simulink model "AariaHIABTorqueR2017a"  (R2017a)
settings: Solver=VariableStepAuto  StartTime=0.0  StopTime=inf  FixedStep=0.1  RelTol=1e-3  EnableMultiTasking=on
model workspace (MATLAB code in the model file):
  | my_a =1;
undefined symbols (not defined in the file or in its folder): AARIAENV, AARIAMAN, AARIASEN, Camera, sensor, Source_TS, X, Y, Z
libraries: sm_lib x350, nesl_utility x205, dspmathops x80, simulink x66, powerlib_meascontrol x3, vrlib x2, aerolibanimutils x1, aerolibutil x1
(part 4 of 9)

== system AariaHIABTorqueR2017a/Subsystem/grab_check_cam above angled down ==
  note: compares spherical coordinates from tool to camera and camera to object (doesn't work always)
  note: compares spherical coordinates from camera to and camera to object
  CamObjSph : Inport
  ObjPose : Inport  Port=2
  TipCamSph : Inport  Port=3
  Logical Operator : Logic  AllPortsSameDT=off  OutDataTypeStr=boolean
  Subsystem : Subsystem
  Sum : Sum
  orientation match : Subsystem  Commented=on
  orientation match1 : Subsystem
  pose match : Subsystem
  grab ok : Outport
  pose ok : Outport  Port=2
  orientation ok : Outport  Port=3
  Bonus : Outport  Port=4  OutDataTypeStr=double
  wires:
  TipCamSph/1 -> orientation match1/1(TipCam)
  Subsystem/1(TipObjPose) -> pose match/1(Obj_pose)
  ObjPose/1 -> Subsystem/1(CamObj)
  CamObjSph/1 -> orientation match1/2(CamObj)
  pose match/1(grab_pose_ok) -> pose ok/1, Logical Operator/1
  Logical Operator/1 -> grab ok/1
  orientation match1/2(Orient_penalty) -> Sum/2
  pose match/2(PoseBonus) -> Sum/1
  Sum/1 -> Bonus/1
  orientation match1/1(Out1) -> orientation ok/1, Logical Operator/2

== system AariaHIABTorqueR2017a/Subsystem2/Subsystem1 ==
  Trigger : TriggerPort  VariantControl=Variant  PortDimensions=1
  Constant : Constant
  Constant1 : Constant  Value=0
  Memory : Memory  InheritSampleTime=on
  Switch : Switch  Criteria=u2 > Threshold
  Out1 : Outport
  wires:
  Constant/1 -> Switch/3
  Switch/1 -> Out1/1, Memory/1
  Memory/1 -> Switch/2
  Constant1/1 -> Switch/1

== system AariaHIABTorqueR2017a/Tool/IMU Tool ==
  Sensor Module1 : Subsystem  mask{nL=nL, nS=1}
      mask prompts: nL "Link Number"; nS "Sensor ID of that link"
      mask DialogControl DescGroupVar Prompt: Virtual IMU
      mask DialogControl DescTextVar Prompt: Measures Connected Body's acceleration and angular velocity in the given point
      mask DialogControl Control2 Prompt: The following numbers defines the corresponding numbers for this sensor to read from the parameters file
  Body Coord : PMIOPort  Port=1  Side=Left
  Reference Coord : PMIOPort  Port=2  Side=Left
  Out1 : Outport
  Out2 : Outport  Port=2
  Out3 : Outport  Port=3
  Out4 : Outport  Port=4
  wires:
  Sensor Module1/3(Out2) -> Out3/1
  Sensor Module1/2(Out4) -> Out2/1
  Sensor Module1/4(Out3) -> Out4/1
  Sensor Module1/1(Out5) -> Out1/1
  connections:
  Sensor Module1/LConn2 -- Reference Coord/RConn1
  Sensor Module1/LConn1 -- Body Coord/RConn1

== system AariaHIABTorqueR2017a/Tool/IMU Tool1 ==
  Sensor Module1 : Subsystem  mask{nL=nL, nS=1}
      mask prompts: nL "Link Number"; nS "Sensor ID of that link"
      mask DialogControl DescGroupVar Prompt: Virtual IMU
      mask DialogControl DescTextVar Prompt: Measures Connected Body's acceleration and angular velocity in the given point
      mask DialogControl Control2 Prompt: The following numbers defines the corresponding numbers for this sensor to read from the parameters file
  Body Coord : PMIOPort  Port=1  Side=Left
  Reference Coord : PMIOPort  Port=2  Side=Left
  Out1 : Outport
  Out2 : Outport  Port=2
  Out3 : Outport  Port=3
  Out4 : Outport  Port=4
  wires:
  Sensor Module1/1(Out5) -> Out1/1
  Sensor Module1/4(Out3) -> Out4/1
  Sensor Module1/2(Out4) -> Out2/1
  Sensor Module1/3(Out2) -> Out3/1
  connections:
  Sensor Module1/LConn1 -- Body Coord/RConn1
  Sensor Module1/LConn2 -- Reference Coord/RConn1

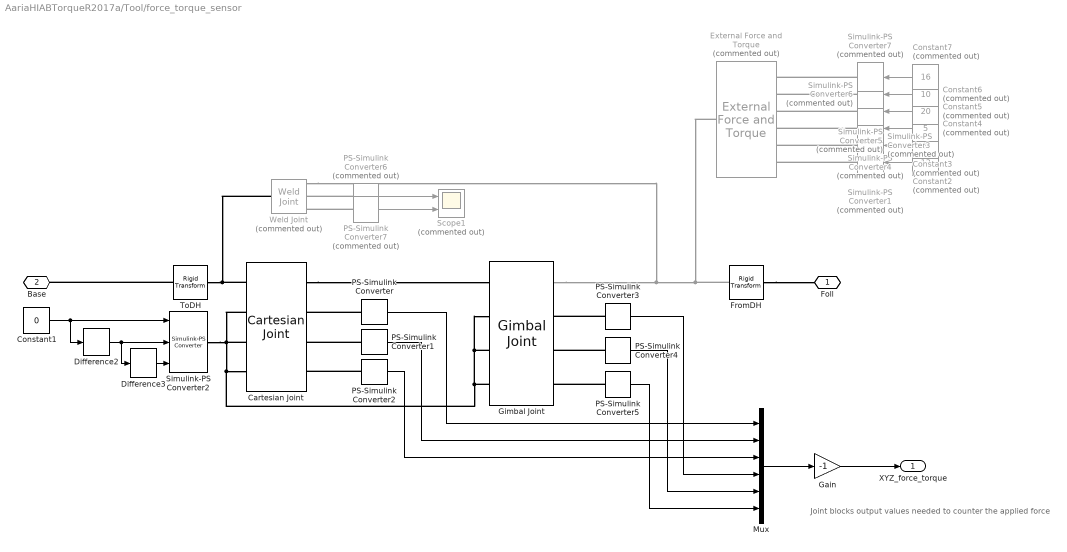
== system AariaHIABTorqueR2017a/Tool/force_torque_sensor ==
  note: Joint blocks output values needed to counter the applied force
  Cartesian Joint : sm_lib/Joints/Cartesian Joint  SenseConstraintForce=off  SenseConstraintForceX=off  SenseConstraintForceY=off  SenseConstraintForceZ=off  SenseConstraintTorque=off  SenseConstraintTorqueX=off  SenseConstraintTorqueY=off  SenseConstraintTorqueZ=off  SenseTotalForce=off  SenseTotalForceX=off  SenseTotalForceY=off  SenseTotalForceZ=off  SenseTotalTorque=off  SenseTotalTorqueX=off  SenseTotalTorqueY=off  SenseTotalTorqueZ=off  CompositeWrenchDir=FollowerOnBase  CompositeWrenchFrame=BaseFrame  PxEquilibriumPosition=0  PxEquilibriumPositionUnits=m  PxSpringStiffness=0  PxSpringStiffnessUnits=N/m  PxDampingCoefficient=0  PxDampingCoefficientUnits=N/(m/s)  PxTorqueActuationMode=ComputedTorque  PxMotionActuationMode=InputMotion  PxSensePosition=off  PxSenseVelocity=off  PxSenseAcceleration=off  PxSenseTorqueForce=on  PxPositionTargetSpecify=off  PxPositionTargetPriority=High  PxPositionTargetValue=0  PxPositionTargetValueUnits=m  PxVelocityTargetSpecify=off  PxVelocityTargetPriority=High  PxVelocityTargetValue=0  PxVelocityTargetValueUnits=m/s  PyEquilibriumPosition=0  PyEquilibriumPositionUnits=m  PySpringStiffness=0  PySpringStiffnessUnits=N/m  PyDampingCoefficient=0  PyDampingCoefficientUnits=N/(m/s)  PyTorqueActuationMode=ComputedTorque  PyMotionActuationMode=InputMotion  PySensePosition=off  PySenseVelocity=off  PySenseAcceleration=off  PySenseTorqueForce=on  PyPositionTargetSpecify=off  PyPositionTargetPriority=High  PyPositionTargetValue=0  PyPositionTargetValueUnits=m  PyVelocityTargetSpecify=off  PyVelocityTargetPriority=High  PyVelocityTargetValue=0  PyVelocityTargetValueUnits=m/s  PzEquilibriumPosition=0  PzEquilibriumPositionUnits=m  PzSpringStiffness=0  PzSpringStiffnessUnits=N/m  PzDampingCoefficient=0  PzDampingCoefficientUnits=N/(m/s)  PzTorqueActuationMode=ComputedTorque  PzMotionActuationMode=InputMotion  PzSensePosition=off  PzSenseVelocity=off  PzSenseAcceleration=off  PzSenseTorqueForce=on  PzPositionTargetSpecify=off  PzPositionTargetPriority=High  PzPositionTargetValue=0  PzPositionTargetValueUnits=m  PzVelocityTargetSpecify=off  PzVelocityTargetPriority=High  PzVelocityTargetValue=0  PzVelocityTargetValueUnits=m/s
  Constant1 : Constant  Value=0
  Constant2 : Constant  Commented=on  Value=13
  Constant3 : Constant  Commented=on
  Constant4 : Constant  Commented=on  Value=5
  Constant5 : Constant  Commented=on  Value=20
  Constant6 : Constant  Commented=on  Value=10
  Constant7 : Constant  Commented=on  Value=16
  Difference2 : simulink/Discrete/Difference  ICPrevInput=0.0  OutMin=[]  OutMax=[]  OutDataType=fixdt(1, 16)  OutScaling=2^-10  DoSatur=off
  Difference3 : simulink/Discrete/Difference  ICPrevInput=0.0  OutMin=[]  OutMax=[]  OutDataType=fixdt(1, 16)  OutScaling=2^-10  DoSatur=off
  External Force and Torque : sm_lib/Forces and Torques/External Force and Torque  Commented=on  ForceResolutionFrame=AttachedFrame  EnableForceX=on  EnableForceY=on  EnableForceZ=on  EnableForce=off  TorqueResolutionFrame=AttachedFrame  EnableTorqueX=on  EnableTorqueY=on  EnableTorqueZ=on  EnableTorque=off
  FromDH : sm_lib/Frames and Transforms/Rigid Transform  TranslationMethod=None  TranslationStandardOffset=0  TranslationLengthUnit=m  TranslationStandardAxis=+Z  TranslationCartesianOffset=[0 0 0]  TranslationROffset=0  TranslationROffsetUnits=m  TranslationZOffset=0  TranslationZOffsetUnits=m  TranslationThetaOffset=0  TranslationThetaOffsetUnits=deg  RotationMethod=RotationMatrix  RotationAngleUnits=deg  RotationStandardAxis=+Z  RotationAngle=0.0  RotationArbitraryAxis=[0 0 1]  FollAlignAxisA=+X  BaseAlignAxisA=+Y  FollAlignAxisB=+Y  BaseAlignAxisB=+Z  RotationSequenceAxes=FollowerAxes  RotationSequence=XYX  RotationSequenceAngles=[0 0 0]  RotationSequenceAnglesUnits=deg  RotationMatrix=AARIAMAN.L(Link_number).toDH'
  Gain : Gain  Gain=-1
  Gimbal Joint : sm_lib/Joints/Gimbal Joint  SenseConstraintForce=off  SenseConstraintForceX=off  SenseConstraintForceY=off  SenseConstraintForceZ=off  SenseConstraintTorque=off  SenseConstraintTorqueX=off  SenseConstraintTorqueY=off  SenseConstraintTorqueZ=off  SenseTotalForce=off  SenseTotalForceX=off  SenseTotalForceY=off  SenseTotalForceZ=off  SenseTotalTorque=off  SenseTotalTorqueX=off  SenseTotalTorqueY=off  SenseTotalTorqueZ=off  CompositeWrenchDir=FollowerOnBase  CompositeWrenchFrame=BaseFrame  RxEquilibriumPosition=0  RxEquilibriumPositionUnits=deg  RxSpringStiffness=0  RxSpringStiffnessUnits=N*m/deg  RxDampingCoefficient=0  RxDampingCoefficientUnits=N*m/(deg/s)  RxTorqueActuationMode=ComputedTorque  RxMotionActuationMode=InputMotion  RxSensePosition=off  RxSenseVelocity=off  RxSenseAcceleration=off  RxSenseTorqueForce=on  RxPositionTargetSpecify=off  RxPositionTargetPriority=High  RxPositionTargetValue=0  RxPositionTargetValueUnits=deg  RxVelocityTargetSpecify=off  RxVelocityTargetPriority=High  RxVelocityTargetValue=0  RxVelocityTargetValueUnits=deg/s  RyEquilibriumPosition=0  RyEquilibriumPositionUnits=deg  RySpringStiffness=0  RySpringStiffnessUnits=N*m/deg  RyDampingCoefficient=0  RyDampingCoefficientUnits=N*m/(deg/s)  RyTorqueActuationMode=ComputedTorque  RyMotionActuationMode=InputMotion  RySensePosition=off  RySenseVelocity=off  RySenseAcceleration=off  RySenseTorqueForce=on  RyPositionTargetSpecify=off  RyPositionTargetPriority=High  RyPositionTargetValue=0  RyPositionTargetValueUnits=deg  RyVelocityTargetSpecify=off  RyVelocityTargetPriority=High  RyVelocityTargetValue=0  RyVelocityTargetValueUnits=deg/s  RzEquilibriumPosition=0  RzEquilibriumPositionUnits=deg  RzSpringStiffness=0  RzSpringStiffnessUnits=N*m/deg  RzDampingCoefficient=0  RzDampingCoefficientUnits=N*m/(deg/s)  RzTorqueActuationMode=ComputedTorque  RzMotionActuationMode=InputMotion  RzSensePosition=off  RzSenseVelocity=off  RzSenseAcceleration=off  RzSenseTorqueForce=on  RzPositionTargetSpecify=off  RzPositionTargetPriority=High  RzPositionTargetValue=0  RzPositionTargetValueUnits=deg  RzVelocityTargetSpecify=off  RzVelocityTargetPriority=High  RzVelocityTargetValue=0  RzVelocityTargetValueUnits=deg/s
      settings: SourceProductName=Simscape Multibody
  Mux : Mux  Inputs=6
  PS-Simulink Converter{,1..5} (6 alike) : nesl_utility/PS-Simulink Converter  PhysicalDomain=network_engine_domain  SubClassName=ps_output  LeftPortType=input  RightPortType=output  PseudoPeriodic=off  Frequencies=[]  Unit=1  AffineConversion=off
  PS-Simulink Converter6 : nesl_utility/PS-Simulink Converter  Commented=on  PhysicalDomain=network_engine_domain  SubClassName=ps_output  LeftPortType=input  RightPortType=output  PseudoPeriodic=off  Frequencies=[]  Unit=1  AffineConversion=off
  PS-Simulink Converter7 : nesl_utility/PS-Simulink Converter  Commented=on  PhysicalDomain=network_engine_domain  SubClassName=ps_output  LeftPortType=input  RightPortType=output  PseudoPeriodic=off  Frequencies=[]  Unit=1  AffineConversion=off
  Scope1 : Scope  Commented=on  NumInputPorts=2
  Simulink-PS Converter{1,3..7} (6 alike) : nesl_utility/Simulink-PS Converter  Commented=on  PhysicalDomain=network_engine_domain  SubClassName=ps_input  LeftPortType=input  RightPortType=output  PseudoPeriodic=off  Frequencies=[]  NoiseDistribution=none  NoiseParameters=[]  Unit=1  AffineConversion=off  FilteringAndDerivatives=provide  SimscapeFilterOrder=1  InputFilterTimeConstant=0.001  UdotUserProvided=0
  Simulink-PS Converter2 : nesl_utility/Simulink-PS Converter  PhysicalDomain=network_engine_domain  SubClassName=ps_input  LeftPortType=input  RightPortType=output  PseudoPeriodic=off  Frequencies=[]  NoiseDistribution=none  NoiseParameters=[]  Unit=1  AffineConversion=off  FilteringAndDerivatives=provide  SimscapeFilterOrder=1  InputFilterTimeConstant=0.001  UdotUserProvided=2
  ToDH : sm_lib/Frames and Transforms/Rigid Transform  TranslationMethod=None  TranslationStandardOffset=0  TranslationLengthUnit=m  TranslationStandardAxis=+Z  TranslationCartesianOffset=[0 0 0]  TranslationROffset=0  TranslationROffsetUnits=m  TranslationZOffset=0  TranslationZOffsetUnits=m  TranslationThetaOffset=0  TranslationThetaOffsetUnits=deg  RotationMethod=RotationMatrix  RotationAngleUnits=deg  RotationStandardAxis=+Z  RotationAngle=0.0  RotationArbitraryAxis=[0 0 1]  FollAlignAxisA=+X  BaseAlignAxisA=+Y  FollAlignAxisB=+Y  BaseAlignAxisB=+Z  RotationSequenceAxes=FollowerAxes  RotationSequence=XYX  RotationSequenceAngles=[0 0 0]  RotationSequenceAnglesUnits=deg  RotationMatrix=AARIAMAN.L(Link_number).toDH
  Weld Joint : sm_lib/Joints/Weld Joint  Commented=on  SenseConstraintForce=on  SenseConstraintForceX=off  SenseConstraintForceY=off  SenseConstraintForceZ=off  SenseConstraintTorque=on  SenseConstraintTorqueX=off  SenseConstraintTorqueY=off  SenseConstraintTorqueZ=off  SenseTotalForce=off  SenseTotalForceX=off  SenseTotalForceY=off  SenseTotalForceZ=off  SenseTotalTorque=off  SenseTotalTorqueX=off  SenseTotalTorqueY=off  SenseTotalTorqueZ=off  CompositeWrenchDir=FollowerOnBase  CompositeWrenchFrame=BaseFrame
  Foll : PMIOPort  Port=1  Side=Right
  Base : PMIOPort  Port=2  Side=Left
  XYZ_force_torque : Outport
  wires:
  Constant1/1 -> Difference2/1, Simulink-PS Converter2/1
  Difference2/1 -> Difference3/1, Simulink-PS Converter2/2
  Difference3/1 -> Simulink-PS Converter2/3
  Constant2/1 -> Simulink-PS Converter1/1
  PS-Simulink Converter/1 -> Mux/1
  PS-Simulink Converter1/1 -> Mux/2
  PS-Simulink Converter2/1 -> Mux/3
  PS-Simulink Converter3/1 -> Mux/4
  PS-Simulink Converter4/1 -> Mux/5
  PS-Simulink Converter5/1 -> Mux/6
  Mux/1 -> Gain/1
  Constant3/1 -> Simulink-PS Converter3/1
  Constant4/1 -> Simulink-PS Converter4/1
  Constant5/1 -> Simulink-PS Converter5/1
  Constant6/1 -> Simulink-PS Converter6/1
  Constant7/1 -> Simulink-PS Converter7/1
  Gain/1 -> XYZ_force_torque/1
  PS-Simulink Converter7/1 -> Scope1/2
  PS-Simulink Converter6/1 -> Scope1/1
  connections:
  Simulink-PS Converter2/RConn1 -- Gimbal Joint/LConn4 -- Gimbal Joint/LConn3 -- Gimbal Joint/LConn2 -- Cartesian Joint/LConn4 -- Cartesian Joint/LConn3 -- Cartesian Joint/LConn2
  PS-Simulink Converter4/LConn1 -- Gimbal Joint/RConn3
  PS-Simulink Converter5/LConn1 -- Gimbal Joint/RConn4
  PS-Simulink Converter3/LConn1 -- Gimbal Joint/RConn2
  ToDH/LConn1 -- Base/RConn1
  PS-Simulink Converter2/LConn1 -- Cartesian Joint/RConn4
  PS-Simulink Converter/LConn1 -- Cartesian Joint/RConn2
  PS-Simulink Converter1/LConn1 -- Cartesian Joint/RConn3
  External Force and Torque/RConn1 -- FromDH/LConn1 -- Weld Joint/RConn1 -- Gimbal Joint/RConn1
  Simulink-PS Converter1/RConn1 -- External Force and Torque/LConn6
  Cartesian Joint/RConn1 -- Gimbal Joint/LConn1
  Cartesian Joint/LConn1 -- ToDH/RConn1 -- Weld Joint/LConn1
  FromDH/RConn1 -- Foll/RConn1
  Simulink-PS Converter3/RConn1 -- External Force and Torque/LConn5
  Simulink-PS Converter4/RConn1 -- External Force and Torque/LConn4
  Simulink-PS Converter5/RConn1 -- External Force and Torque/LConn3
  Simulink-PS Converter6/RConn1 -- External Force and Torque/LConn2
  Simulink-PS Converter7/RConn1 -- External Force and Torque/LConn1
  PS-Simulink Converter6/LConn1 -- Weld Joint/RConn2
  PS-Simulink Converter7/LConn1 -- Weld Joint/RConn3

== system AariaHIABTorqueR2017a/Tool Sensors/Camera sensor ==
  Gain : Gain  Gain=0
  Mux : Mux  Inputs=3
  Mux1 : Mux  Inputs=3
  PS-Simulink Converter{2..8} (7 alike) : nesl_utility/PS-Simulink Converter  PhysicalDomain=network_engine_domain  SubClassName=ps_output  LeftPortType=input  RightPortType=output  PseudoPeriodic=off  Frequencies=[]  Unit=1  AffineConversion=off
  Sum1 : Sum  Inputs=|++
  Sum2 : Sum  Inputs=++|
  Sum3 : Sum  Inputs=++|
  Transform Sensor : sm_lib/Frames and Transforms/Transform Sensor  MeasurementFrame=Base  SenseAngle=off  SenseAxis=off  SenseAngle1=off  SenseAngle2=off  SenseAngle3=off  SenseQ=off  SenseR=on  SenseOmegaX=off  SenseOmegaY=off  SenseOmegaZ=off  SenseOmega1=off  SenseOmega2=off  SenseOmega3=off  SenseQDot=off  SenseRDot=off  SenseAlphaX=off  SenseAlphaY=off  SenseAlphaZ=off  SenseAlpha1=off  SenseAlpha2=off  SenseAlpha3=off  SenseQDDot=off  SenseRDDot=off  SenseX=on  SenseY=on  SenseZ=on  SenseRad=off  SenseAzim=on  SenseDist=on  SenseInc=on  SenseXDot=off  SenseYDot=off  SenseZDot=off  SenseRadDot=off  SenseAzimDot=off  SenseDistDot=off  SenseIncDot=off  SenseXDDot=off  SenseYDDot=off  SenseZDDot=off  SenseRadDDot=off  SenseAzimDDot=off  SenseDistDDot=off  SenseIncDDot=off
  coord_sens : sm_lib/Body Elements/Graphic  GraphicType=Marker  MarkerShape=Frame  MarkerSize=AARIAMAN.vis.coord_sizeS  GraphicVisPropType=SimpleVisualProperties  GraphicDiffuseColor=AARIAMAN.vis.col_s  GraphicSpecularColor=[0.5 0.5 0.5 1.0]  GraphicAmbientColor=[0.15 0.15 0.15 1.0]  GraphicEmissiveColor=[0.0 0.0 0.0 1.0]  GraphicShininess=75  GraphicOpacity=AARIAMAN.vis.opacity_s
      settings: SourceProductName=Simscape Multibody
  omega_noise : Subsystem  Commented=on
  placeholder noise 3 : Subsystem
  placeholder noise1 : Subsystem
  placeholder noise2 : Subsystem
  Body Frame : PMIOPort  Port=1  Side=Left
  Reference Frame : PMIOPort  Port=2  Side=Left
  Out3 : Outport
  Out1 : Outport  Port=2
  Out2 : Outport  Port=3
  wires:
  Sum2/1 -> Out1/1  "cartesian"
  PS-Simulink Converter8/1 -> Sum3/2  "R_actual"
  PS-Simulink Converter7/1 -> Mux1/3
  PS-Simulink Converter5/1 -> Mux1/1
  PS-Simulink Converter6/1 -> Mux1/2
  Mux/1 -> Sum2/2  "cartesian"
  PS-Simulink Converter4/1 -> Mux/3
  PS-Simulink Converter2/1 -> Mux/1
  PS-Simulink Converter3/1 -> Mux/2
  Mux1/1 -> Sum1/1  "spherical"
  Sum3/1 -> Out3/1  "rotation"
  placeholder noise2/1(noise) -> Sum3/1
  placeholder noise 3/1(noise) -> Gain/1
  Sum1/1 -> Out2/1  "spherical"
  placeholder noise1/1(noise) -> Sum2/1
  Gain/1 -> Sum1/2
  connections:
  Transform Sensor/RConn7 -- PS-Simulink Converter6/LConn1
  Transform Sensor/RConn8 -- PS-Simulink Converter7/LConn1
  PS-Simulink Converter8/LConn1 -- Transform Sensor/RConn2
  Transform Sensor/RConn6 -- PS-Simulink Converter5/LConn1
  Transform Sensor/RConn5 -- PS-Simulink Converter4/LConn1
  Transform Sensor/LConn1 -- Reference Frame/RConn1
  Transform Sensor/RConn4 -- PS-Simulink Converter3/LConn1
  Transform Sensor/RConn3 -- PS-Simulink Converter2/LConn1
  coord_sens/RConn1 -- Body Frame/RConn1 -- Transform Sensor/RConn1

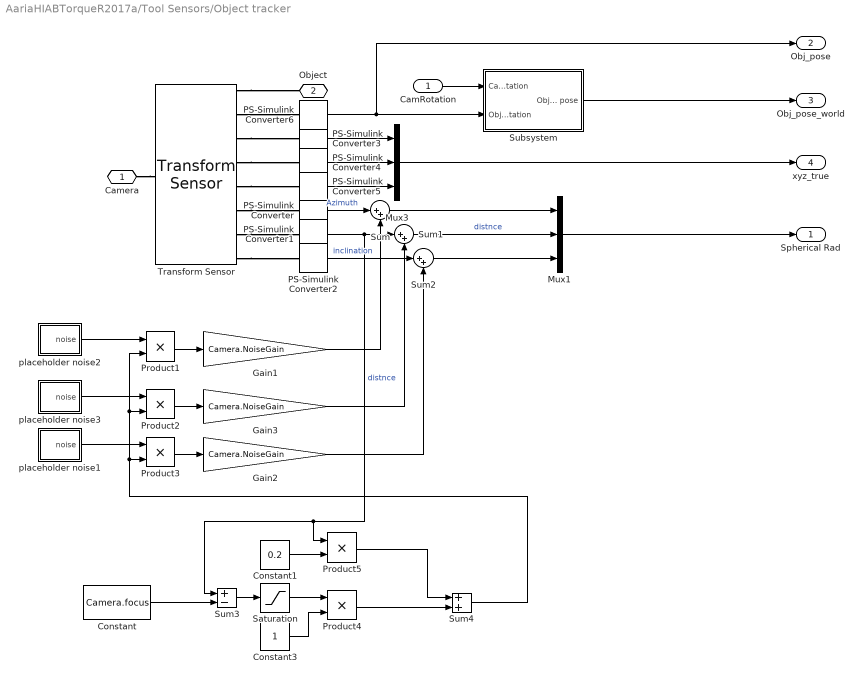
== system AariaHIABTorqueR2017a/Tool Sensors/Object tracker ==
  CamRotation : Inport
  Constant : Constant  Value=Camera.focus
  Constant1 : Constant  Value=0.2
  Constant3 : Constant
  Gain1 : Gain  Gain=Camera.NoiseGain
  Gain2 : Gain  Gain=Camera.NoiseGain
  Gain3 : Gain  Gain=Camera.NoiseGain
  Mux1 : Mux  Inputs=3
  Mux3 : Mux  Inputs=3
  PS-Simulink Converter{,1..6} (7 alike) : nesl_utility/PS-Simulink Converter  PhysicalDomain=network_engine_domain  SubClassName=ps_output  LeftPortType=input  RightPortType=output  PseudoPeriodic=off  Frequencies=[]  Unit=1  AffineConversion=off
  Product{1..5} (5 alike) : Product
  Saturation : Saturate  UpperLimit=20  LowerLimit=0
  Subsystem : Subsystem
  Sum : Sum  Inputs=|++
  Sum1 : Sum  Inputs=|++
  Sum2 : Sum  Inputs=|++
  Sum3 : Sum  Inputs=+|-
  Sum4 : Sum
  "Transform Sensor " : sm_lib/Frames and Transforms/Transform Sensor  MeasurementFrame=Base  SenseAngle=off  SenseAxis=off  SenseAngle1=off  SenseAngle2=off  SenseAngle3=off  SenseQ=off  SenseR=on  SenseOmegaX=off  SenseOmegaY=off  SenseOmegaZ=off  SenseOmega1=off  SenseOmega2=off  SenseOmega3=off  SenseQDot=off  SenseRDot=off  SenseAlphaX=off  SenseAlphaY=off  SenseAlphaZ=off  SenseAlpha1=off  SenseAlpha2=off  SenseAlpha3=off  SenseQDDot=off  SenseRDDot=off  SenseX=on  SenseY=on  SenseZ=on  SenseRad=off  SenseAzim=on  SenseDist=on  SenseInc=on  SenseXDot=off  SenseYDot=off  SenseZDot=off  SenseRadDot=off  SenseAzimDot=off  SenseDistDot=off  SenseIncDot=off  SenseXDDot=off  SenseYDDot=off  SenseZDDot=off  SenseRadDDot=off  SenseAzimDDot=off  SenseDistDDot=off  SenseIncDDot=off
  placeholder noise1 : Subsystem
  placeholder noise2 : Subsystem
  placeholder noise3 : Subsystem
  Camera : PMIOPort  Port=1  Side=Left
  Object : PMIOPort  Port=2  Side=Right
  Spherical Rad : Outport
  Obj_pose : Outport  Port=2
  Obj_pose_world : Outport  Port=3
  xyz_true : Outport  Port=4
  wires:
  Sum1/1 -> Mux1/2  "distnce"
  Mux1/1 -> Spherical Rad/1
  placeholder noise1/1(noise) -> Product3/1
  PS-Simulink Converter/1 -> Sum/1  "Azimuth"
  Sum/1 -> Mux1/1
  PS-Simulink Converter2/1 -> Sum2/1  "inclination"
  Sum2/1 -> Mux1/3
  placeholder noise2/1(noise) -> Product1/1
  PS-Simulink Converter1/1 -> Sum3/1, Product5/1, Sum1/1  "distnce"
  placeholder noise3/1(noise) -> Product2/1
  Gain3/1 -> Sum1/2
  Gain1/1 -> Sum/2
  PS-Simulink Converter3/1 -> Mux3/1
  PS-Simulink Converter4/1 -> Mux3/2
  PS-Simulink Converter5/1 -> Mux3/3
  Mux3/1 -> xyz_true/1
  Gain2/1 -> Sum2/2
  CamRotation/1 -> Subsystem/1(Camera rotation)
  Subsystem/1(Object world pose) -> Obj_pose_world/1
  PS-Simulink Converter6/1 -> Obj_pose/1, Subsystem/2(Object rotation)
  Constant/1 -> Sum3/2
  Constant1/1 -> Product5/2
  Product4/1 -> Sum4/2
  Product1/1 -> Gain1/1
  Product2/1 -> Gain3/1
  Product3/1 -> Gain2/1
  Sum4/1 -> Product1/2, Product2/2, Product3/2
  Sum3/1 -> Saturation/1
  Saturation/1 -> Product4/1
  Constant3/1 -> Product4/2
  Product5/1 -> Sum4/1
  connections:
  Camera/RConn1 -- "Transform Sensor "/LConn1
  "Transform Sensor "/RConn1 -- Object/RConn1
  "Transform Sensor "/RConn8 -- PS-Simulink Converter2/LConn1
  "Transform Sensor "/RConn7 -- PS-Simulink Converter1/LConn1
  "Transform Sensor "/RConn6 -- PS-Simulink Converter/LConn1
  "Transform Sensor "/RConn5 -- PS-Simulink Converter5/LConn1
  "Transform Sensor "/RConn4 -- PS-Simulink Converter4/LConn1
  "Transform Sensor "/RConn3 -- PS-Simulink Converter3/LConn1
  "Transform Sensor "/RConn2 -- PS-Simulink Converter6/LConn1

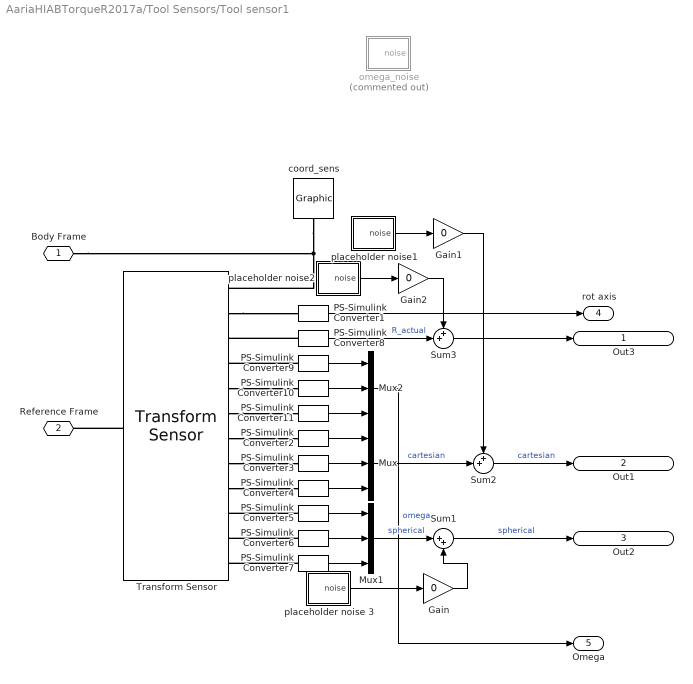
== system AariaHIABTorqueR2017a/Tool Sensors/Tool sensor1 ==
  Gain : Gain  Gain=0
  Gain1 : Gain  Gain=0
  Gain2 : Gain  Gain=0
  Mux : Mux  Inputs=3
  Mux1 : Mux  Inputs=3
  Mux2 : Mux  Inputs=3
  PS-Simulink Converter{1..11} (11 alike) : nesl_utility/PS-Simulink Converter  PhysicalDomain=network_engine_domain  SubClassName=ps_output  LeftPortType=input  RightPortType=output  PseudoPeriodic=off  Frequencies=[]  Unit=1  AffineConversion=off
  Sum1 : Sum  Inputs=|++
  Sum2 : Sum  Inputs=++|
  Sum3 : Sum  Inputs=++|
  Transform Sensor : sm_lib/Frames and Transforms/Transform Sensor  MeasurementFrame=Base  SenseAngle=off  SenseAxis=on  SenseAngle1=off  SenseAngle2=off  SenseAngle3=off  SenseQ=off  SenseR=on  SenseOmegaX=on  SenseOmegaY=on  SenseOmegaZ=on  SenseOmega1=off  SenseOmega2=off  SenseOmega3=off  SenseQDot=off  SenseRDot=off  SenseAlphaX=off  SenseAlphaY=off  SenseAlphaZ=off  SenseAlpha1=off  SenseAlpha2=off  SenseAlpha3=off  SenseQDDot=off  SenseRDDot=off  SenseX=on  SenseY=on  SenseZ=on  SenseRad=off  SenseAzim=on  SenseDist=on  SenseInc=on  SenseXDot=off  SenseYDot=off  SenseZDot=off  SenseRadDot=off  SenseAzimDot=off  SenseDistDot=off  SenseIncDot=off  SenseXDDot=off  SenseYDDot=off  SenseZDDot=off  SenseRadDDot=off  SenseAzimDDot=off  SenseDistDDot=off  SenseIncDDot=off
  coord_sens : sm_lib/Body Elements/Graphic  GraphicType=Marker  MarkerShape=Frame  MarkerSize=AARIAMAN.vis.coord_sizeS  GraphicVisPropType=SimpleVisualProperties  GraphicDiffuseColor=AARIAMAN.vis.col_s  GraphicSpecularColor=[0.5 0.5 0.5 1.0]  GraphicAmbientColor=[0.15 0.15 0.15 1.0]  GraphicEmissiveColor=[0.0 0.0 0.0 1.0]  GraphicShininess=75  GraphicOpacity=AARIAMAN.vis.opacity_s
      settings: SourceProductName=Simscape Multibody
  omega_noise : Subsystem  Commented=on
  placeholder noise 3 : Subsystem
  placeholder noise1 : Subsystem
  placeholder noise2 : Subsystem
  Body Frame : PMIOPort  Port=1  Side=Left
  Reference Frame : PMIOPort  Port=2  Side=Left
  Out3 : Outport
  Out1 : Outport  Port=2
  Out2 : Outport  Port=3
  rot axis : Outport  Port=4
  Omega : Outport  Port=5
  wires:
  Sum2/1 -> Out1/1  "cartesian"
  PS-Simulink Converter8/1 -> Sum3/2  "R_actual"
  PS-Simulink Converter7/1 -> Mux1/3
  PS-Simulink Converter5/1 -> Mux1/1
  PS-Simulink Converter6/1 -> Mux1/2
  Mux/1 -> Sum2/2  "cartesian"
  PS-Simulink Converter4/1 -> Mux/3
  PS-Simulink Converter2/1 -> Mux/1
  PS-Simulink Converter3/1 -> Mux/2
  Mux1/1 -> Sum1/1  "spherical"
  placeholder noise2/1(noise) -> Gain2/1
  placeholder noise 3/1(noise) -> Gain/1
  Sum1/1 -> Out2/1  "spherical"
  placeholder noise1/1(noise) -> Gain1/1
  Gain/1 -> Sum1/2
  PS-Simulink Converter1/1 -> rot axis/1
  Gain1/1 -> Sum2/1
  Gain2/1 -> Sum3/1
  Sum3/1 -> Out3/1
  PS-Simulink Converter10/1 -> Mux2/2
  PS-Simulink Converter9/1 -> Mux2/1
  PS-Simulink Converter11/1 -> Mux2/3
  Mux2/1 -> Omega/1  "omega"
  connections:
  PS-Simulink Converter8/LConn1 -- Transform Sensor/RConn3
  Transform Sensor/RConn9 -- PS-Simulink Converter4/LConn1
  Transform Sensor/LConn1 -- Reference Frame/RConn1
  Transform Sensor/RConn8 -- PS-Simulink Converter3/LConn1
  Transform Sensor/RConn7 -- PS-Simulink Converter2/LConn1
  coord_sens/RConn1 -- Body Frame/RConn1 -- Transform Sensor/RConn1
  PS-Simulink Converter5/LConn1 -- Transform Sensor/RConn10
  PS-Simulink Converter6/LConn1 -- Transform Sensor/RConn11
  PS-Simulink Converter7/LConn1 -- Transform Sensor/RConn12
  Transform Sensor/RConn2 -- PS-Simulink Converter1/LConn1
  PS-Simulink Converter9/LConn1 -- Transform Sensor/RConn4
  Transform Sensor/RConn5 -- PS-Simulink Converter10/LConn1
  Transform Sensor/RConn6 -- PS-Simulink Converter11/LConn1

== system AariaHIABTorqueR2017a/Tool Sensors/Tool sensor2 ==
  Gain : Gain  Gain=0
  Mux : Mux  Inputs=3
  Mux1 : Mux  Inputs=3
  PS-Simulink Converter{2..8} (7 alike) : nesl_utility/PS-Simulink Converter  PhysicalDomain=network_engine_domain  SubClassName=ps_output  LeftPortType=input  RightPortType=output  PseudoPeriodic=off  Frequencies=[]  Unit=1  AffineConversion=off
  Sum1 : Sum  Inputs=|++
  Sum2 : Sum  Inputs=++|
  Sum3 : Sum  Inputs=++|
  Transform Sensor : sm_lib/Frames and Transforms/Transform Sensor  MeasurementFrame=Base  SenseAngle=off  SenseAxis=off  SenseAngle1=off  SenseAngle2=off  SenseAngle3=off  SenseQ=off  SenseR=on  SenseOmegaX=off  SenseOmegaY=off  SenseOmegaZ=off  SenseOmega1=off  SenseOmega2=off  SenseOmega3=off  SenseQDot=off  SenseRDot=off  SenseAlphaX=off  SenseAlphaY=off  SenseAlphaZ=off  SenseAlpha1=off  SenseAlpha2=off  SenseAlpha3=off  SenseQDDot=off  SenseRDDot=off  SenseX=on  SenseY=on  SenseZ=on  SenseRad=off  SenseAzim=on  SenseDist=on  SenseInc=on  SenseXDot=off  SenseYDot=off  SenseZDot=off  SenseRadDot=off  SenseAzimDot=off  SenseDistDot=off  SenseIncDot=off  SenseXDDot=off  SenseYDDot=off  SenseZDDot=off  SenseRadDDot=off  SenseAzimDDot=off  SenseDistDDot=off  SenseIncDDot=off
  coord_sens : sm_lib/Body Elements/Graphic  GraphicType=Marker  MarkerShape=Frame  MarkerSize=AARIAMAN.vis.coord_sizeS  GraphicVisPropType=SimpleVisualProperties  GraphicDiffuseColor=AARIAMAN.vis.col_s  GraphicSpecularColor=[0.5 0.5 0.5 1.0]  GraphicAmbientColor=[0.15 0.15 0.15 1.0]  GraphicEmissiveColor=[0.0 0.0 0.0 1.0]  GraphicShininess=75  GraphicOpacity=AARIAMAN.vis.opacity_s
      settings: SourceProductName=Simscape Multibody
  placeholder noise 3 : Subsystem
  placeholder noise1 : Subsystem
  placeholder noise2 : Subsystem
  Body Frame : PMIOPort  Port=1  Side=Left
  Reference Frame : PMIOPort  Port=2  Side=Left
  Out3 : Outport
  Out1 : Outport  Port=2
  Out2 : Outport  Port=3
  wires:
  Gain/1 -> Sum1/2
  placeholder noise1/1(noise) -> Sum2/1
  Sum1/1 -> Out2/1  "spherical"
  placeholder noise 3/1(noise) -> Gain/1
  placeholder noise2/1(noise) -> Sum3/1
  Sum3/1 -> Out3/1  "rotation"
  Mux1/1 -> Sum1/1  "spherical"
  PS-Simulink Converter3/1 -> Mux/2
  PS-Simulink Converter2/1 -> Mux/1
  PS-Simulink Converter4/1 -> Mux/3
  Mux/1 -> Sum2/2  "cartesian"
  PS-Simulink Converter6/1 -> Mux1/2
  PS-Simulink Converter5/1 -> Mux1/1
  PS-Simulink Converter7/1 -> Mux1/3
  PS-Simulink Converter8/1 -> Sum3/2  "R_actual"
  Sum2/1 -> Out1/1  "cartesian"
  connections:
  PS-Simulink Converter7/LConn1 -- Transform Sensor/RConn8
  PS-Simulink Converter6/LConn1 -- Transform Sensor/RConn7
  PS-Simulink Converter5/LConn1 -- Transform Sensor/RConn6
  Transform Sensor/RConn1 -- Body Frame/RConn1 -- coord_sens/RConn1
  Transform Sensor/RConn3 -- PS-Simulink Converter2/LConn1
  Transform Sensor/RConn4 -- PS-Simulink Converter3/LConn1
  Transform Sensor/LConn1 -- Reference Frame/RConn1
  Transform Sensor/RConn5 -- PS-Simulink Converter4/LConn1
  PS-Simulink Converter8/LConn1 -- Transform Sensor/RConn2

== system AariaHIABTorqueR2017a/Base/BaseVSS/BaseEmpty ==
  IMU Base : Subsystem  mask{nL=Link_number}
      mask prompts: nL "Link Number (nL)"
      mask DialogControl DescTextVar Prompt: A Set of IMUs for one body
  Mux1 : Mux  Inputs=2
  Terminator : Terminator
  Terminator1 : Terminator
  Start : PMIOPort  Port=1  Side=Left
  End : PMIOPort  Port=2  Side=Right
  IMU : Outport
  wires:
  IMU Base/4(Out4) -> Terminator1/1
  IMU Base/1(Out1) -> Mux1/1
  IMU Base/2(Out2) -> Mux1/2
  Mux1/1 -> IMU/1
  IMU Base/3(Out3) -> Terminator/1
  connections:
  Start/RConn1 -- IMU Base/LConn2 -- IMU Base/LConn1 -- End/RConn1

== system AariaHIABTorqueR2017a/Base/BaseVSS/BaseMotion ==
  Cartesian Joint : sm_lib/Joints/Cartesian Joint  SenseConstraintForce=off  SenseConstraintForceX=off  SenseConstraintForceY=off  SenseConstraintForceZ=off  SenseConstraintTorque=off  SenseConstraintTorqueX=off  SenseConstraintTorqueY=off  SenseConstraintTorqueZ=off  SenseTotalForce=off  SenseTotalForceX=off  SenseTotalForceY=off  SenseTotalForceZ=off  SenseTotalTorque=off  SenseTotalTorqueX=off  SenseTotalTorqueY=off  SenseTotalTorqueZ=off  CompositeWrenchDir=FollowerOnBase  CompositeWrenchFrame=BaseFrame  PxEquilibriumPosition=0  PxEquilibriumPositionUnits=m  PxSpringStiffness=0  PxSpringStiffnessUnits=N/m  PxDampingCoefficient=AARIAMAN.D.prismaticdamping  PxDampingCoefficientUnits=N/(m/s)  PxTorqueActuationMode=ComputedTorque  PxMotionActuationMode=InputMotion  PxSensePosition=off  PxSenseVelocity=off  PxSenseAcceleration=off  PxSenseTorqueForce=off  PxPositionTargetSpecify=off  PxPositionTargetPriority=High  PxPositionTargetValue=0  PxPositionTargetValueUnits=m  PxVelocityTargetSpecify=off  PxVelocityTargetPriority=High  PxVelocityTargetValue=0  PxVelocityTargetValueUnits=m/s  PyEquilibriumPosition=0  PyEquilibriumPositionUnits=m  PySpringStiffness=0  PySpringStiffnessUnits=N/m  PyDampingCoefficient=0  PyDampingCoefficientUnits=N/(m/s)  PyTorqueActuationMode=ComputedTorque  PyMotionActuationMode=InputMotion  PySensePosition=off  PySenseVelocity=off  PySenseAcceleration=off  PySenseTorqueForce=off  PyPositionTargetSpecify=off  PyPositionTargetPriority=High  PyPositionTargetValue=0  PyPositionTargetValueUnits=m  PyVelocityTargetSpecify=off  PyVelocityTargetPriority=High  PyVelocityTargetValue=0  PyVelocityTargetValueUnits=m/s  PzEquilibriumPosition=0  PzEquilibriumPositionUnits=m  PzSpringStiffness=0  PzSpringStiffnessUnits=N/m  PzDampingCoefficient=0  PzDampingCoefficientUnits=N/(m/s)  PzTorqueActuationMode=ComputedTorque  PzMotionActuationMode=InputMotion  PzSensePosition=off  PzSenseVelocity=off  PzSenseAcceleration=off  PzSenseTorqueForce=off  PzPositionTargetSpecify=off  PzPositionTargetPriority=High  PzPositionTargetValue=0  PzPositionTargetValueUnits=m  PzVelocityTargetSpecify=off  PzVelocityTargetPriority=High  PzVelocityTargetValue=0  PzVelocityTargetValueUnits=m/s
  Gimbal Joint : sm_lib/Joints/Gimbal Joint  SenseConstraintForce=off  SenseConstraintForceX=off  SenseConstraintForceY=off  SenseConstraintForceZ=off  SenseConstraintTorque=off  SenseConstraintTorqueX=off  SenseConstraintTorqueY=off  SenseConstraintTorqueZ=off  SenseTotalForce=off  SenseTotalForceX=off  SenseTotalForceY=off  SenseTotalForceZ=off  SenseTotalTorque=off  SenseTotalTorqueX=off  SenseTotalTorqueY=off  SenseTotalTorqueZ=off  CompositeWrenchDir=FollowerOnBase  CompositeWrenchFrame=BaseFrame  RxEquilibriumPosition=0  RxEquilibriumPositionUnits=deg  RxSpringStiffness=0  RxSpringStiffnessUnits=N*m/deg  RxDampingCoefficient=AARIAMAN.D.revolutedamping  RxDampingCoefficientUnits=N*m/(deg/s)  RxTorqueActuationMode=ComputedTorque  RxMotionActuationMode=InputMotion  RxSensePosition=off  RxSenseVelocity=off  RxSenseAcceleration=off  RxSenseTorqueForce=off  RxPositionTargetSpecify=off  RxPositionTargetPriority=High  RxPositionTargetValue=0  RxPositionTargetValueUnits=deg  RxVelocityTargetSpecify=off  RxVelocityTargetPriority=High  RxVelocityTargetValue=0  RxVelocityTargetValueUnits=deg/s  RyEquilibriumPosition=0  RyEquilibriumPositionUnits=deg  RySpringStiffness=0  RySpringStiffnessUnits=N*m/deg  RyDampingCoefficient=0  RyDampingCoefficientUnits=N*m/(deg/s)  RyTorqueActuationMode=ComputedTorque  RyMotionActuationMode=InputMotion  RySensePosition=off  RySenseVelocity=off  RySenseAcceleration=off  RySenseTorqueForce=off  RyPositionTargetSpecify=off  RyPositionTargetPriority=High  RyPositionTargetValue=0  RyPositionTargetValueUnits=deg  RyVelocityTargetSpecify=off  RyVelocityTargetPriority=High  RyVelocityTargetValue=0  RyVelocityTargetValueUnits=deg/s  RzEquilibriumPosition=0  RzEquilibriumPositionUnits=deg  RzSpringStiffness=0  RzSpringStiffnessUnits=N*m/deg  RzDampingCoefficient=0  RzDampingCoefficientUnits=N*m/(deg/s)  RzTorqueActuationMode=ComputedTorque  RzMotionActuationMode=InputMotion  RzSensePosition=off  RzSenseVelocity=off  RzSenseAcceleration=off  RzSenseTorqueForce=off  RzPositionTargetSpecify=off  RzPositionTargetPriority=High  RzPositionTargetValue=0  RzPositionTargetValueUnits=deg  RzVelocityTargetSpecify=off  RzVelocityTargetPriority=High  RzVelocityTargetValue=0  RzVelocityTargetValueUnits=deg/s
      settings: SourceProductName=Simscape Multibody
  IMU Base : Subsystem  mask{nL=Link_number}
      mask prompts: nL "Link Number (nL)"
      mask DialogControl DescTextVar Prompt: A Set of IMUs for one body
  Mux : Mux  Inputs=2
  Sine Wave2 : Sin  Amplitude=AARIAMAN.B.trans.ampx  Bias=AARIAMAN.B.trans.biasx  Frequency=AARIAMAN.B.trans.freqx  Phase=AARIAMAN.B.trans.phasex  SampleTime=AARIAENV.Source_TS
  Sine Wave3 : Sin  Amplitude=AARIAMAN.B.trans.ampy  Bias=AARIAMAN.B.trans.biasy  Frequency=AARIAMAN.B.trans.freqy  Phase=AARIAMAN.B.trans.phasey  SampleTime=AARIAENV.Source_TS
  Sine Wave4 : Sin  Amplitude=AARIAMAN.B.trans.ampz  Bias=AARIAMAN.B.trans.biasz  Frequency=AARIAMAN.B.trans.freqz  Phase=AARIAMAN.B.trans.phasez  SampleTime=AARIAENV.Source_TS
  Sine Wave5 : Sin  Amplitude=AARIAMAN.B.rot.ampx  Bias=AARIAMAN.B.rot.biasx  Frequency=AARIAMAN.B.rot.freqx  Phase=AARIAMAN.B.rot.phasex  SampleTime=AARIAENV.Source_TS
  Sine Wave6 : Sin  Amplitude=AARIAMAN.B.rot.ampy  Bias=AARIAMAN.B.rot.biasy  Frequency=AARIAMAN.B.rot.freqy  Phase=AARIAMAN.B.rot.phasey  SampleTime=AARIAENV.Source_TS
  Sine Wave7 : Sin  Amplitude=AARIAMAN.B.rot.ampz  Bias=AARIAMAN.B.rot.biasz  Frequency=AARIAMAN.B.rot.freqz  Phase=AARIAMAN.B.rot.phasez  SampleTime=AARIAENV.Source_TS
  Terminator : Terminator
  Terminator1 : Terminator
  x 2motion2 : Subsystem
  x 2motion3 : Subsystem
  x 2motion4 : Subsystem
  x 2motion5 : Subsystem
  x 2motion6 : Subsystem
  x 2motion7 : Subsystem
  Start : PMIOPort  Port=1  Side=Left
  End : PMIOPort  Port=2  Side=Right
  IMU : Outport
  wires:
  Sine Wave7/1 -> x 2motion7/1(X)
  Sine Wave6/1 -> x 2motion6/1(X)
  Sine Wave5/1 -> x 2motion5/1(X)
  Sine Wave3/1 -> x 2motion3/1(X)
  IMU Base/3(Out3) -> Terminator/1
  IMU Base/1(Out1) -> Mux/1
  IMU Base/2(Out2) -> Mux/2
  Sine Wave4/1 -> x 2motion4/1(X)
  Mux/1 -> IMU/1
  IMU Base/4(Out4) -> Terminator1/1
  Sine Wave2/1 -> x 2motion2/1(X)
  connections:
  x 2motion7/RConn1 -- Gimbal Joint/LConn4
  x 2motion5/RConn1 -- Gimbal Joint/LConn2
  Cartesian Joint/RConn1 -- Gimbal Joint/LConn1
  x 2motion6/RConn1 -- Gimbal Joint/LConn3
  x 2motion4/RConn1 -- Cartesian Joint/LConn4
  x 2motion2/RConn1 -- Cartesian Joint/LConn2
  x 2motion3/RConn1 -- Cartesian Joint/LConn3
  IMU Base/LConn2 -- Cartesian Joint/LConn1 -- Start/RConn1
  IMU Base/LConn1 -- Gimbal Joint/RConn1 -- End/RConn1

== system AariaHIABTorqueR2017a/Base/BaseVSS/BaseTorque ==
  Cartesian Joint : sm_lib/Joints/Cartesian Joint  SenseConstraintForce=off  SenseConstraintForceX=off  SenseConstraintForceY=off  SenseConstraintForceZ=off  SenseConstraintTorque=off  SenseConstraintTorqueX=off  SenseConstraintTorqueY=off  SenseConstraintTorqueZ=off  SenseTotalForce=off  SenseTotalForceX=off  SenseTotalForceY=off  SenseTotalForceZ=off  SenseTotalTorque=off  SenseTotalTorqueX=off  SenseTotalTorqueY=off  SenseTotalTorqueZ=off  CompositeWrenchDir=FollowerOnBase  CompositeWrenchFrame=BaseFrame  PxEquilibriumPosition=0  PxEquilibriumPositionUnits=m  PxSpringStiffness=0  PxSpringStiffnessUnits=N/m  PxDampingCoefficient=AARIAMAN.D.prismaticdamping  PxDampingCoefficientUnits=N/(m/s)  PxTorqueActuationMode=InputTorque  PxMotionActuationMode=ComputedMotion  PxSensePosition=off  PxSenseVelocity=off  PxSenseAcceleration=off  PxSenseTorqueForce=off  PxPositionTargetSpecify=off  PxPositionTargetPriority=High  PxPositionTargetValue=0  PxPositionTargetValueUnits=m  PxVelocityTargetSpecify=off  PxVelocityTargetPriority=High  PxVelocityTargetValue=0  PxVelocityTargetValueUnits=m/s  PyEquilibriumPosition=0  PyEquilibriumPositionUnits=m  PySpringStiffness=0  PySpringStiffnessUnits=N/m  PyDampingCoefficient=0  PyDampingCoefficientUnits=N/(m/s)  PyTorqueActuationMode=ComputedTorque  PyMotionActuationMode=InputMotion  PySensePosition=off  PySenseVelocity=off  PySenseAcceleration=off  PySenseTorqueForce=off  PyPositionTargetSpecify=off  PyPositionTargetPriority=High  PyPositionTargetValue=0  PyPositionTargetValueUnits=m  PyVelocityTargetSpecify=off  PyVelocityTargetPriority=High  PyVelocityTargetValue=0  PyVelocityTargetValueUnits=m/s  PzEquilibriumPosition=0  PzEquilibriumPositionUnits=m  PzSpringStiffness=0  PzSpringStiffnessUnits=N/m  PzDampingCoefficient=0  PzDampingCoefficientUnits=N/(m/s)  PzTorqueActuationMode=ComputedTorque  PzMotionActuationMode=InputMotion  PzSensePosition=off  PzSenseVelocity=off  PzSenseAcceleration=off  PzSenseTorqueForce=off  PzPositionTargetSpecify=off  PzPositionTargetPriority=High  PzPositionTargetValue=0  PzPositionTargetValueUnits=m  PzVelocityTargetSpecify=off  PzVelocityTargetPriority=High  PzVelocityTargetValue=0  PzVelocityTargetValueUnits=m/s
  Gimbal Joint : sm_lib/Joints/Gimbal Joint  SenseConstraintForce=off  SenseConstraintForceX=off  SenseConstraintForceY=off  SenseConstraintForceZ=off  SenseConstraintTorque=off  SenseConstraintTorqueX=off  SenseConstraintTorqueY=off  SenseConstraintTorqueZ=off  SenseTotalForce=off  SenseTotalForceX=off  SenseTotalForceY=off  SenseTotalForceZ=off  SenseTotalTorque=off  SenseTotalTorqueX=off  SenseTotalTorqueY=off  SenseTotalTorqueZ=off  CompositeWrenchDir=FollowerOnBase  CompositeWrenchFrame=BaseFrame  RxEquilibriumPosition=0  RxEquilibriumPositionUnits=deg  RxSpringStiffness=0  RxSpringStiffnessUnits=N*m/deg  RxDampingCoefficient=AARIAMAN.D.revolutedamping  RxDampingCoefficientUnits=N*m/(deg/s)  RxTorqueActuationMode=InputTorque  RxMotionActuationMode=ComputedMotion  RxSensePosition=off  RxSenseVelocity=off  RxSenseAcceleration=off  RxSenseTorqueForce=off  RxPositionTargetSpecify=off  RxPositionTargetPriority=High  RxPositionTargetValue=0  RxPositionTargetValueUnits=deg  RxVelocityTargetSpecify=off  RxVelocityTargetPriority=High  RxVelocityTargetValue=0  RxVelocityTargetValueUnits=deg/s  RyEquilibriumPosition=0  RyEquilibriumPositionUnits=deg  RySpringStiffness=0  RySpringStiffnessUnits=N*m/deg  RyDampingCoefficient=0  RyDampingCoefficientUnits=N*m/(deg/s)  RyTorqueActuationMode=ComputedTorque  RyMotionActuationMode=InputMotion  RySensePosition=off  RySenseVelocity=off  RySenseAcceleration=off  RySenseTorqueForce=off  RyPositionTargetSpecify=off  RyPositionTargetPriority=High  RyPositionTargetValue=0  RyPositionTargetValueUnits=deg  RyVelocityTargetSpecify=off  RyVelocityTargetPriority=High  RyVelocityTargetValue=0  RyVelocityTargetValueUnits=deg/s  RzEquilibriumPosition=0  RzEquilibriumPositionUnits=deg  RzSpringStiffness=0  RzSpringStiffnessUnits=N*m/deg  RzDampingCoefficient=0  RzDampingCoefficientUnits=N*m/(deg/s)  RzTorqueActuationMode=ComputedTorque  RzMotionActuationMode=InputMotion  RzSensePosition=off  RzSenseVelocity=off  RzSenseAcceleration=off  RzSenseTorqueForce=off  RzPositionTargetSpecify=off  RzPositionTargetPriority=High  RzPositionTargetValue=0  RzPositionTargetValueUnits=deg  RzVelocityTargetSpecify=off  RzVelocityTargetPriority=High  RzVelocityTargetValue=0  RzVelocityTargetValueUnits=deg/s
      settings: SourceProductName=Simscape Multibody
  IMU Base : Subsystem  mask{nL=Link_number}
      mask prompts: nL "Link Number (nL)"
      mask DialogControl DescTextVar Prompt: A Set of IMUs for one body
  Mux : Mux  Inputs=2
  Sine Wave2 : Sin  Amplitude=AARIAMAN.B.trans.tampx  Bias=AARIAMAN.B.trans.tbiasx  Frequency=AARIAMAN.B.trans.tfreqx  Phase=AARIAMAN.B.trans.tphasex  SampleTime=AARIAENV.Source_TS
  Sine Wave3 : Sin  Amplitude=AARIAMAN.B.trans.tampy  Bias=AARIAMAN.B.trans.tbiasy  Frequency=AARIAMAN.B.trans.tfreqy  Phase=AARIAMAN.B.trans.tphasey  SampleTime=AARIAENV.Source_TS
  Sine Wave4 : Sin  Amplitude=AARIAMAN.B.trans.tampz  Bias=AARIAMAN.B.trans.tbiasz  Frequency=AARIAMAN.B.trans.tfreqz  Phase=AARIAMAN.B.trans.tphasez  SampleTime=AARIAENV.Source_TS
  Sine Wave5 : Sin  Amplitude=AARIAMAN.B.rot.tampx  Bias=AARIAMAN.B.rot.tbiasx  Frequency=AARIAMAN.B.rot.tfreqx  Phase=AARIAMAN.B.rot.tphasex  SampleTime=AARIAENV.Source_TS
  Sine Wave6 : Sin  Amplitude=AARIAMAN.B.rot.tampy  Bias=AARIAMAN.B.rot.tbiasy  Frequency=AARIAMAN.B.rot.tfreqy  Phase=AARIAMAN.B.rot.tphasey  SampleTime=AARIAENV.Source_TS
  Sine Wave7 : Sin  Amplitude=AARIAMAN.B.rot.tampz  Bias=AARIAMAN.B.rot.tbiasz  Frequency=AARIAMAN.B.rot.tfreqz  Phase=AARIAMAN.B.rot.tphasez  SampleTime=AARIAENV.Source_TS
  Terminator : Terminator
  Terminator1 : Terminator
  x 2motion2 : Subsystem
  x 2motion3 : Subsystem
  x 2motion4 : Subsystem
  x 2motion5 : Subsystem
  x 2motion6 : Subsystem
  x 2motion7 : Subsystem
  Start : PMIOPort  Port=1  Side=Left
  End : PMIOPort  Port=2  Side=Right
  IMU : Outport
  wires:
  Sine Wave5/1 -> x 2motion5/1(X)
  Sine Wave6/1 -> x 2motion6/1(X)
  Sine Wave3/1 -> x 2motion3/1(X)
  Sine Wave7/1 -> x 2motion7/1(X)
  IMU Base/3(Out3) -> Terminator/1
  IMU Base/1(Out1) -> Mux/1
  IMU Base/2(Out2) -> Mux/2
  Sine Wave4/1 -> x 2motion4/1(X)
  Mux/1 -> IMU/1
  IMU Base/4(Out4) -> Terminator1/1
  Sine Wave2/1 -> x 2motion2/1(X)
  connections:
  x 2motion7/RConn1 -- Gimbal Joint/LConn4
  x 2motion5/RConn1 -- Gimbal Joint/LConn2
  Cartesian Joint/RConn1 -- Gimbal Joint/LConn1
  x 2motion6/RConn1 -- Gimbal Joint/LConn3
  x 2motion4/RConn1 -- Cartesian Joint/LConn4
  x 2motion2/RConn1 -- Cartesian Joint/LConn2
  x 2motion3/RConn1 -- Cartesian Joint/LConn3
  IMU Base/LConn2 -- Cartesian Joint/LConn1 -- Start/RConn1
  IMU Base/LConn1 -- Gimbal Joint/RConn1 -- End/RConn1

== system AariaHIABTorqueR2017a/Joint1/RevoluteMotion/IMU Sensors ==
  Sensor Module1 : Subsystem  mask{nL=nL, nS=1}
      mask prompts: nL "Link Number"; nS "Sensor ID of that link"
      mask DialogControl DescGroupVar Prompt: Virtual IMU
      mask DialogControl DescTextVar Prompt: Measures Connected Body's acceleration and angular velocity in the given point
      mask DialogControl Control2 Prompt: The following numbers defines the corresponding numbers for this sensor to read from the parameters file
  Sensor Module2 : Subsystem  mask{nL=nL, nS=2}
      mask prompts: nL "Link Number"; nS "Sensor ID of that link"
      mask DialogControl DescGroupVar Prompt: Virtual IMU
      mask DialogControl DescTextVar Prompt: Measures Connected Body's acceleration and angular velocity in the given point
      mask DialogControl Control2 Prompt: The following numbers defines the corresponding numbers for this sensor to read from the parameters file
  Terminator{,1..3} (4 alike) : Terminator
  Body Coord : PMIOPort  Port=1  Side=Left
  Reference Coord : PMIOPort  Port=2  Side=Left
  Out1 : Outport
  Out2 : Outport  Port=2
  Out5 : Outport  Port=3
  Out6 : Outport  Port=4
  wires:
  Sensor Module2/3(Out2) -> Terminator2/1
  Sensor Module2/1(Out5) -> Out5/1
  Sensor Module2/4(Out3) -> Terminator3/1
  Sensor Module2/2(Out4) -> Out6/1
  Sensor Module1/1(Out5) -> Out1/1
  Sensor Module1/4(Out3) -> Terminator1/1
  Sensor Module1/2(Out4) -> Out2/1
  Sensor Module1/3(Out2) -> Terminator/1
  connections:
  Sensor Module1/LConn1 -- Body Coord/RConn1 -- Sensor Module2/LConn1
  Sensor Module1/LConn2 -- Reference Coord/RConn1 -- Sensor Module2/LConn2

== system AariaHIABTorqueR2017a/Joint1/RevoluteMotion/x 2motion ==
  X : Inport
  Simulink-PS Converter : nesl_utility/Simulink-PS Converter  PhysicalDomain=network_engine_domain  SubClassName=ps_input  LeftPortType=input  RightPortType=output  PseudoPeriodic=off  Frequencies=[]  NoiseDistribution=none  NoiseParameters=[]  Unit=1  AffineConversion=off  FilteringAndDerivatives=provide  SimscapeFilterOrder=1  InputFilterTimeConstant=0.001  UdotUserProvided=2
  Unit Delay : UnitDelay  SampleTime=-1
  Unit Delay1 : UnitDelay  SampleTime=-1
  Motion for PS : PMIOPort  Port=1  Side=Right
  wires:
  X/1 -> Unit Delay/1, Simulink-PS Converter/1
  Unit Delay/1 -> Unit Delay1/1, Simulink-PS Converter/2
  Unit Delay1/1 -> Simulink-PS Converter/3
  connections:
  Simulink-PS Converter/RConn1 -- Motion for PS/RConn1

== system AariaHIABTorqueR2017a/Joint2/RevoluteMotion/IMU Sensors ==
  Sensor Module1 : Subsystem  mask{nL=nL, nS=1}
      mask prompts: nL "Link Number"; nS "Sensor ID of that link"
      mask DialogControl DescGroupVar Prompt: Virtual IMU
      mask DialogControl DescTextVar Prompt: Measures Connected Body's acceleration and angular velocity in the given point
      mask DialogControl Control2 Prompt: The following numbers defines the corresponding numbers for this sensor to read from the parameters file
  Sensor Module2 : Subsystem  mask{nL=nL, nS=2}
      mask prompts: nL "Link Number"; nS "Sensor ID of that link"
      mask DialogControl DescGroupVar Prompt: Virtual IMU
      mask DialogControl DescTextVar Prompt: Measures Connected Body's acceleration and angular velocity in the given point
      mask DialogControl Control2 Prompt: The following numbers defines the corresponding numbers for this sensor to read from the parameters file
  Terminator{,1..3} (4 alike) : Terminator
  Body Coord : PMIOPort  Port=1  Side=Left
  Reference Coord : PMIOPort  Port=2  Side=Left
  Out1 : Outport
  Out2 : Outport  Port=2
  Out5 : Outport  Port=3
  Out6 : Outport  Port=4
  wires:
  Sensor Module2/3(Out2) -> Terminator2/1
  Sensor Module2/1(Out5) -> Out5/1
  Sensor Module2/4(Out3) -> Terminator3/1
  Sensor Module2/2(Out4) -> Out6/1
  Sensor Module1/1(Out5) -> Out1/1
  Sensor Module1/4(Out3) -> Terminator1/1
  Sensor Module1/2(Out4) -> Out2/1
  Sensor Module1/3(Out2) -> Terminator/1
  connections:
  Sensor Module1/LConn1 -- Body Coord/RConn1 -- Sensor Module2/LConn1
  Sensor Module1/LConn2 -- Reference Coord/RConn1 -- Sensor Module2/LConn2

== system AariaHIABTorqueR2017a/Joint2/RevoluteMotion/x 2motion ==
  X : Inport
  Simulink-PS Converter : nesl_utility/Simulink-PS Converter  PhysicalDomain=network_engine_domain  SubClassName=ps_input  LeftPortType=input  RightPortType=output  PseudoPeriodic=off  Frequencies=[]  NoiseDistribution=none  NoiseParameters=[]  Unit=1  AffineConversion=off  FilteringAndDerivatives=provide  SimscapeFilterOrder=1  InputFilterTimeConstant=0.001  UdotUserProvided=0
  Motion for PS : PMIOPort  Port=1  Side=Right
  wires:
  X/1 -> Simulink-PS Converter/1
  connections:
  Simulink-PS Converter/RConn1 -- Motion for PS/RConn1

== system AariaHIABTorqueR2017a/Joint3/RevoluteMotion/IMU Sensors ==
  Sensor Module1 : Subsystem  mask{nL=nL, nS=1}
      mask prompts: nL "Link Number"; nS "Sensor ID of that link"
      mask DialogControl DescGroupVar Prompt: Virtual IMU
      mask DialogControl DescTextVar Prompt: Measures Connected Body's acceleration and angular velocity in the given point
      mask DialogControl Control2 Prompt: The following numbers defines the corresponding numbers for this sensor to read from the parameters file
  Sensor Module2 : Subsystem  mask{nL=nL, nS=2}
      mask prompts: nL "Link Number"; nS "Sensor ID of that link"
      mask DialogControl DescGroupVar Prompt: Virtual IMU
      mask DialogControl DescTextVar Prompt: Measures Connected Body's acceleration and angular velocity in the given point
      mask DialogControl Control2 Prompt: The following numbers defines the corresponding numbers for this sensor to read from the parameters file
  Terminator{,1..3} (4 alike) : Terminator
  Body Coord : PMIOPort  Port=1  Side=Left
  Reference Coord : PMIOPort  Port=2  Side=Left
  Out1 : Outport
  Out2 : Outport  Port=2
  Out5 : Outport  Port=3
  Out6 : Outport  Port=4
  wires:
  Sensor Module2/3(Out2) -> Terminator2/1
  Sensor Module2/1(Out5) -> Out5/1
  Sensor Module2/4(Out3) -> Terminator3/1
  Sensor Module2/2(Out4) -> Out6/1
  Sensor Module1/1(Out5) -> Out1/1
  Sensor Module1/4(Out3) -> Terminator1/1
  Sensor Module1/2(Out4) -> Out2/1
  Sensor Module1/3(Out2) -> Terminator/1
  connections:
  Sensor Module1/LConn1 -- Body Coord/RConn1 -- Sensor Module2/LConn1
  Sensor Module1/LConn2 -- Reference Coord/RConn1 -- Sensor Module2/LConn2

== system AariaHIABTorqueR2017a/Joint3/RevoluteMotion/x 2motion ==
  X : Inport
  Simulink-PS Converter : nesl_utility/Simulink-PS Converter  PhysicalDomain=network_engine_domain  SubClassName=ps_input  LeftPortType=input  RightPortType=output  PseudoPeriodic=off  Frequencies=[]  NoiseDistribution=none  NoiseParameters=[]  Unit=1  AffineConversion=off  FilteringAndDerivatives=provide  SimscapeFilterOrder=1  InputFilterTimeConstant=0.001  UdotUserProvided=0
  Motion for PS : PMIOPort  Port=1  Side=Right
  wires:
  X/1 -> Simulink-PS Converter/1
  connections:
  Simulink-PS Converter/RConn1 -- Motion for PS/RConn1
